simulink model "usb2dynamixel_demo"  (Simulink 7.7)
settings: Solver=FixedStepDiscrete  StartTime=0.0  StopTime=10.0  RelTol=1e-3
undefined symbols (not defined in the file): usb2dynamixel_communication_setup
libraries: lib_darwinop x5
settings Model: Creator=florent  LastModifiedBy=eleve
settings DataIOCC: SignalLoggingSaveFormat=Dataset
settings OptimizationCC: ExpressionDepthLimit=128
settings DebuggingCC: FcnCallInpInsideContextMsg=Enable All
settings CodeAppCC: CustomSymbolStrType=$N$R$M_T
settings GRTTargetCC: CombineOutputUpdateFcns=on

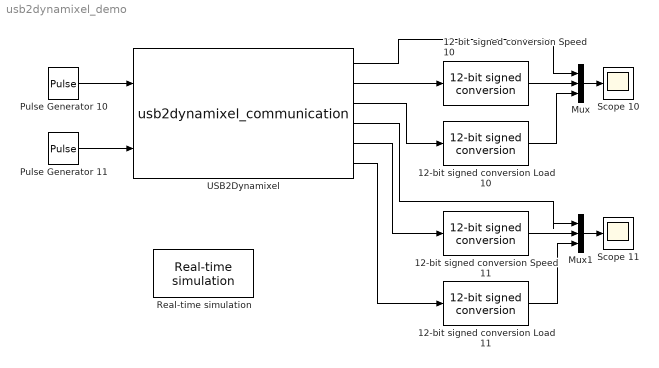
== system usb2dynamixel_demo ==
  12-bit signed conversion Load 10 : lib_darwinop/12-bit signed conversion
  12-bit signed conversion Load 11 : lib_darwinop/12-bit signed conversion
  12-bit signed conversion Speed 10 : lib_darwinop/12-bit signed conversion
  12-bit signed conversion Speed 11 : lib_darwinop/12-bit signed conversion
  Mux : Mux  Inputs=3
  Mux1 : Mux  Inputs=3
  Pulse Generator 10 : DiscretePulseGenerator  PulseType=Time based  Amplitude=800  Period=5  PulseWidth=50
  Pulse Generator 11 : DiscretePulseGenerator  PulseType=Time based  Amplitude=800  Period=3  PulseWidth=50
  Real-time simulation : lib_darwinop/Real-time simulation  TimeScalingFactor=1
  Scope 10 : Scope
  Scope 11 : Scope
      settings: YMin=-1250  YMax=1000
  USB2Dynamixel : M-S-Function  StartFcn=usb2dynamixel_communication_setup('StartFcn');  StopFcn=usb2dynamixel_communication_setup('StopFcn');  FunctionName=usb2dynamixel_communication  Parameters=COMPort,BaudRate,SampleTime,Frame,ReadIndex,WriteIndex,DisableStatusReturn  mask{COMPort='COM11', BaudRate=1000000, SampleTime=0.05, Frame=[ 2 10 36 6 3 10 30 2 0 0 2 11 36 6 3 11 30 2 0 0], ReadIndex=[ 1 2;3 2;5 2;7 2;9 2;11 2], WriteIndex=[ 9 2;19 2], DisableStatusReturn=0}
      settings: DeleteFcn=usb2dynamixel_communication_setup('DeleteFcn');  ModelCloseFcn=usb2dynamixel_communication_setup('ModelCloseFcn');  NameChangeFcn=usb2dynamixel_communication_setup('NameChangeFcn');  OpenFcn=usb2dynamixel_communication_setup('OpenFcn');
      mask Display:
      | image(imread('usb2dynamixel.jpg'))
      | 
      | port_label('output',1,'RX24F(10)/Position')
      | port_label('output',2,'RX24F(10)/Speed')
      | port_label('output',3,'RX24F(10)/Load')
      | port_label('output',4,'RX24F(11)/Position')
      | port_label('output',5,'RX24F(11)/Speed')
      | port_label('output',6,'RX24F(11)/Load')
      | 
      | port_label('input',1,'RX24F(10)/Goal Position')
      | port_label('input',2,'RX24F(11)/Goal Position')
  wires:
  USB2Dynamixel/2 -> 12-bit signed conversion Speed 10/1
  USB2Dynamixel/3 -> 12-bit signed conversion Load 10/1
  USB2Dynamixel/5 -> 12-bit signed conversion Speed 11/1
  USB2Dynamixel/6 -> 12-bit signed conversion Load 11/1
  12-bit signed conversion Speed 10/1 -> Mux/2
  12-bit signed conversion Load 10/1 -> Mux/3
  USB2Dynamixel/1 -> Mux/1
  12-bit signed conversion Speed 11/1 -> Mux1/2
  USB2Dynamixel/4 -> Mux1/1
  12-bit signed conversion Load 11/1 -> Mux1/3
  Mux/1 -> Scope 10/1
  Mux1/1 -> Scope 11/1
  Pulse Generator 10/1 -> USB2Dynamixel/1
  Pulse Generator 11/1 -> USB2Dynamixel/2
